simulink model "proc"  (R2023b)
settings: Solver=VariableStepAuto  StartTime=0.0  StopTime=inf  RelTol=1e-3
settings Model: Creator=votua  LastModifiedBy=votua

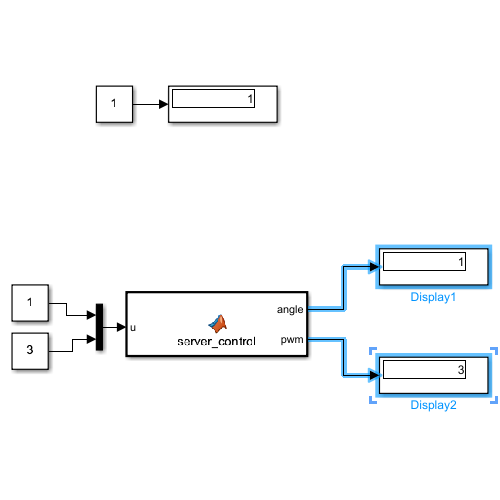
[thumbnail: Simulink's stored preview of the top-level diagram]
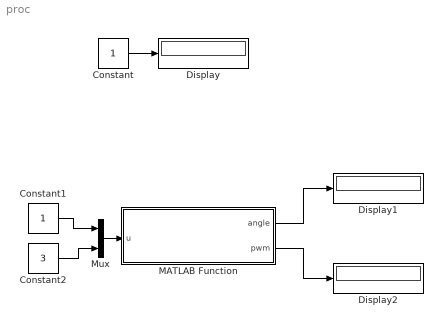
== system proc ==
  Constant : Constant
  Constant1 : Constant
  Constant2 : Constant  Value=3
  Display : Display
  Display1 : Display
  Display2 : Display
  MATLAB Function : MATLAB Function  TreatAsAtomicUnit=on
  Mux : Mux  Inputs=2
  wires:
  Constant/1 -> Display/1
  MATLAB Function/1(angle) -> Display1/1
  MATLAB Function/2(pwm) -> Display2/1
  Mux/1 -> MATLAB Function/1(u)
  Constant1/1 -> Mux/1
  Constant2/1 -> Mux/2

== matlab function proc/MATLAB Function ==
  data: u input; angle output; pwm output
function [angle,pwm] = server_control(u)
    angle = u(1);
    pwm = u(2);
    
    data = string(pwm) + ' ' + string(angle);

    write(server, data, "uint8");  
end
